simulink model "Nonlinear_momentum_wheel_model"  (R2019a)
settings: Solver=ode5  StartTime=0.0  StopTime=t  FixedStep=dt  RelTol=1e-3
values from neighbouring files (symbols this model uses):
  alpha_x = MGX    (= 5e-09)    [SCUBED_ADACS.m]
  alpha_y = MGY    (= 5e-09)    [SCUBED_ADACS.m]
  alpha_z = MGY    (= 5e-09)    [SCUBED_ADACS.m]
  C_I = 1 + A/2 + 2*J/I    (= 2.016)    [SCUBED_ADACS.m]
  C_II = 1 + B/2 + 2*J/I    (= 2.0105)    [SCUBED_ADACS.m]
  C_III = 1 + C/2 + 2*J/I    (= 2.023)    [SCUBED_ADACS.m]
  J_I = (B-C)/I    (= -12.5)    [SCUBED_ADACS.m]
  J_II = (C-A)/I    (= 7)    [SCUBED_ADACS.m]
  J_III = (A-B)/I    (= 5.5)    [SCUBED_ADACS.m]
  MGX = Mgx/I    (= 5e-09)    [SCUBED_ADACS.m]
  MGY = Mgy/I    (= 5e-09)    [SCUBED_ADACS.m]
  MGZ = Mgz/I    (= 0.05)    [SCUBED_ADACS.m]
  omega_x = MGX    (= 5e-09)    [SCUBED_ADACS.m]    (also in test_case_1.m = 1.99098659277e-07)
  omega_y = MGY    (= 5e-09)    [SCUBED_ADACS.m]
  omega_z = MGY    (= 5e-09)    [SCUBED_ADACS.m]
settings Model: PauseTimes=2900000  Creator=jepar  LastModifiedBy=jepar

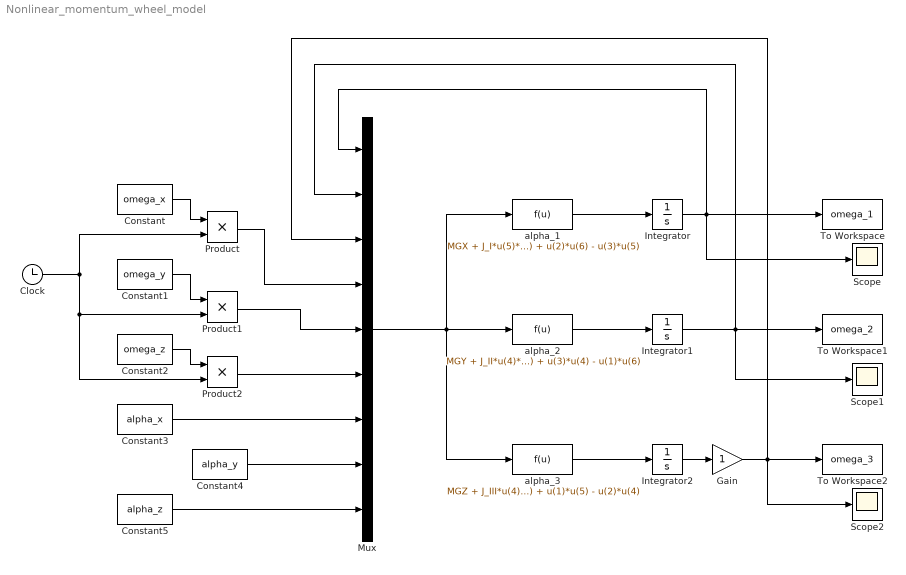
== system Nonlinear_momentum_wheel_model ==
  Clock : Clock
  Constant : Constant  Value=omega_x
  Constant1 : Constant  Value=omega_y
  Constant2 : Constant  Value=omega_z
  Constant3 : Constant  Value=alpha_x
  Constant4 : Constant  Value=alpha_y
  Constant5 : Constant  Value=alpha_z
  Gain : Gain
  Integrator : Integrator
  Integrator1 : Integrator
  Integrator2 : Integrator
  Mux : Mux  Inputs=9
  Product : Product
  Product1 : Product
  Product2 : Product
  Scope : Scope
  Scope1 : Scope
  Scope2 : Scope
  To Workspace : ToWorkspace  VariableName=omega_1  SaveFormat=Structure With Time  SampleTime=-1
  To Workspace1 : ToWorkspace  VariableName=omega_2  SaveFormat=Structure With Time  SampleTime=-1
  To Workspace2 : ToWorkspace  VariableName=omega_3  SaveFormat=Structure With Time  SampleTime=-1
  alpha_1 : Fcn  Expr=MGX + J_I*u(5)*u(6) - C_I*u(7) + u(2)*u(6) - u(3)*u(5)
  alpha_2 : Fcn  Expr=MGY + J_II*u(4)*u(6) - C_II*u(8) + u(3)*u(4) - u(1)*u(6)
  alpha_3 : Fcn  Expr=MGZ + J_III*u(4)*u(5) - C_III*u(9) + u(1)*u(5) - u(2)*u(4)
  wires:
  Integrator1/1 -> To Workspace1/1, Scope1/1, Mux/2
  Constant3/1 -> Mux/7
  Constant4/1 -> Mux/8
  Constant5/1 -> Mux/9
  alpha_1/1 -> Integrator/1
  alpha_2/1 -> Integrator1/1
  alpha_3/1 -> Integrator2/1
  Mux/1 -> alpha_3/1, alpha_1/1, alpha_2/1
  Integrator/1 -> To Workspace/1, Scope/1, Mux/1
  Integrator2/1 -> Gain/1
  Constant/1 -> Product/1
  Product/1 -> Mux/4
  Clock/1 -> Product2/2, Product1/2, Product/2
  Constant1/1 -> Product1/1
  Constant2/1 -> Product2/1
  Product1/1 -> Mux/5
  Product2/1 -> Mux/6
  Gain/1 -> To Workspace2/1, Scope2/1, Mux/3
